simulink model "part1_WORKS"  (R2018b)
settings: Solver=FixedStepAuto  StartTime=0.0  StopTime=10.0  FixedStep=1e-3  RelTol=1e-3  EnableMultiTasking=on
undefined symbols (not defined in the file): A0, A1, D0, D1, D10, D11, D12, D13, D2, D3, D4, D5, D6, D7, D8, D9, PTA0, PTA1, PTA2, PTB2, PTB23, PTB3, PTB9, PTC16, PTC17, PTC2, PTC3, PTC4, PTD0, PTD1, PTD2, PTD3
libraries: frdmk64flib x26, xpcutilitieslib x9
settings Model: ExtModeTrigDuration=5  Creator=Buggs  LastModifiedBy=siddharthravichandran
settings OptimizationCC: PassReuseOutputArgsAs=Individual arguments  MaxStackSize=64
settings DebuggingCC: ParameterTunabilityLossMsg=error
settings HardwareCC: ProdBitPerPointer=32  ProdBitPerSizeT=32  ProdBitPerPtrDiffT=32  ProdLargestAtomicInteger=Long  ProdLargestAtomicFloat=Double  ProdWordSize=32  ProdHWDeviceType=ARM Compatible->ARM Cortex
settings SFSimCC: MATLABDynamicMemAlloc=off
settings RTWCC: SystemTargetFile=ert.tlc  HardwareBoard=NXP FRDM-K64F  TLCOptions="-aInlineSetEventsForThisBaseRateFcn=TLC_FALSE -aSuppressMultiTaskScheduler=TLC_FALSE  -aRateBasedStepFcn=0"  TemplateMakefile=ert_default_tmf  GenerateReport=on  Toolchain=GNU Tools for ARM Embedded Processors  IncludeHyperlinkInReport=on  LaunchReport=on  GenerateTraceInfo=on  GenerateTraceReport=on  GenerateTraceReportSl=on  GenerateTraceReportSf=on  GenerateTraceReportEml=on
settings CodeAppCC: ForceParamTrailComments=on  IgnoreCustomStorageClasses=off  OperatorAnnotations=on  SimulinkDataObjDesc=on  SFDataObjDesc=on  InsertBlockDesc=on

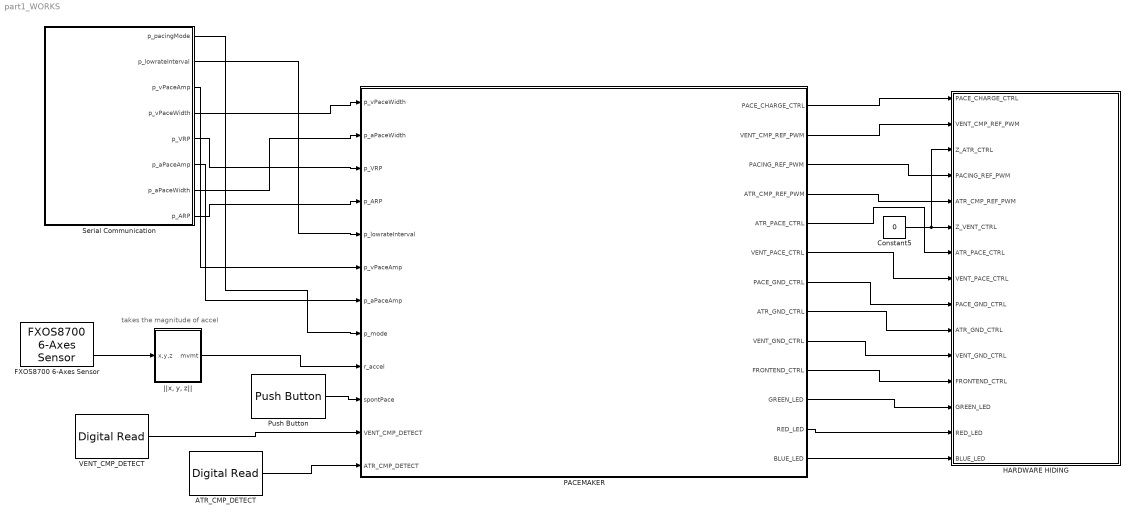
== system part1_WORKS ==
  note: takes the magnitude of accel
  ATR_CMP_DETECT : frdmk64flib/Digital Read  Whichpin=PTC16 (D0)  SampleTime=-1
      settings: SourceProductName=Simulink Coder Support Package for NXP FRDM-K64F Board
  Constant5 : Constant  Value=0  OutDataTypeStr=boolean
  FXOS8700 6-Axes Sensor : frdmk64flib/FXOS8700 6-Axes Sensor  Activesensor=Accelerometer and Magnetometer  ODR=800Hz  HybridODR=400Hz  Accelfullrange=-4g to +4g  SampleTime=-1
      settings: SourceProductName=Simulink Coder Support Package for NXP FRDM-K64F Board
  "HARDWARE HIDING " : Subsystem
  PACEMAKER : Stateflow chart  TreatAsAtomicUnit=on
  Push Button : frdmk64flib/Push Button  Whichswitch=SW2  SampleTime1=-1
      settings: SourceProductName=Simulink Coder Support Package for NXP FRDM-K64F Board
  Serial Communication : Subsystem
  VENT_CMP_DETECT : frdmk64flib/Digital Read  Whichpin=PTC17 (D1)  SampleTime=-1
      settings: SourceProductName=Simulink Coder Support Package for NXP FRDM-K64F Board
  "||x, y, z||" : Subsystem
  wires:
  FXOS8700 6-Axes Sensor/2 -> "||x, y, z||"/1(x,y,z)
  "||x, y, z||"/1(mvmt) -> PACEMAKER/9(r_accel)
  Serial Communication/2(p_lowrateInterval) -> PACEMAKER/5(p_lowrateInterval)
  Serial Communication/1(p_pacingMode) -> PACEMAKER/8(p_mode)
  Push Button/1 -> PACEMAKER/10(spontPace)
  VENT_CMP_DETECT/1 -> PACEMAKER/11(VENT_CMP_DETECT)
  ATR_CMP_DETECT/1 -> PACEMAKER/12(ATR_CMP_DETECT)
  PACEMAKER/11(GREEN_LED) -> "HARDWARE HIDING "/13(GREEN_LED)
  PACEMAKER/10(FRONTEND_CTRL) -> "HARDWARE HIDING "/12(FRONTEND_CTRL)
  PACEMAKER/4(ATR_CMP_REF_PWM) -> "HARDWARE HIDING "/5(ATR_CMP_REF_PWM)
  Constant5/1 -> "HARDWARE HIDING "/3(Z_ATR_CTRL), "HARDWARE HIDING "/6(Z_VENT_CTRL)
  PACEMAKER/1(PACE_CHARGE_CTRL) -> "HARDWARE HIDING "/1(PACE_CHARGE_CTRL)
  PACEMAKER/2(VENT_CMP_REF_PWM) -> "HARDWARE HIDING "/2(VENT_CMP_REF_PWM)
  PACEMAKER/7(PACE_GND_CTRL) -> "HARDWARE HIDING "/9(PACE_GND_CTRL)
  PACEMAKER/9(VENT_GND_CTRL) -> "HARDWARE HIDING "/11(VENT_GND_CTRL)
  PACEMAKER/6(VENT_PACE_CTRL) -> "HARDWARE HIDING "/8(VENT_PACE_CTRL)
  PACEMAKER/8(ATR_GND_CTRL) -> "HARDWARE HIDING "/10(ATR_GND_CTRL)
  PACEMAKER/5(ATR_PACE_CTRL) -> "HARDWARE HIDING "/7(ATR_PACE_CTRL)
  PACEMAKER/3(PACING_REF_PWM) -> "HARDWARE HIDING "/4(PACING_REF_PWM)
  PACEMAKER/12(RED_LED) -> "HARDWARE HIDING "/14(RED_LED)
  PACEMAKER/13(BLUE_LED) -> "HARDWARE HIDING "/15(BLUE_LED)
  Serial Communication/5(p_VRP) -> PACEMAKER/3(p_VRP)
  Serial Communication/8(p_ARP) -> PACEMAKER/4(p_ARP)
  Serial Communication/4(p_vPaceWidth) -> PACEMAKER/1(p_vPaceWidth)
  Serial Communication/7(p_aPaceWidth) -> PACEMAKER/2(p_aPaceWidth)
  Serial Communication/3(p_vPaceAmp) -> PACEMAKER/6(p_vPaceAmp)
  Serial Communication/6(p_aPaceAmp) -> PACEMAKER/7(p_aPaceAmp)

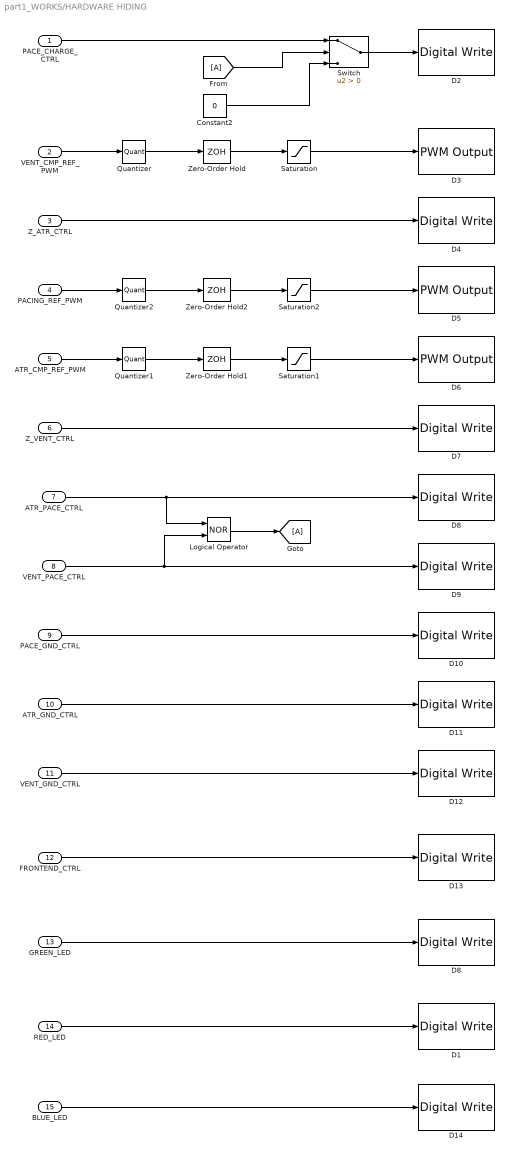
== system part1_WORKS/HARDWARE HIDING  ==
  PACE_CHARGE_CTRL : Inport  OutDataTypeStr=boolean
  VENT_CMP_REF_PWM : Inport  Port=2  OutDataTypeStr=double
  Z_ATR_CTRL : Inport  Port=3  OutDataTypeStr=boolean
  PACING_REF_PWM : Inport  Port=4  OutDataTypeStr=double
  ATR_CMP_REF_PWM : Inport  Port=5  OutDataTypeStr=double
  Z_VENT_CTRL : Inport  Port=6  OutDataTypeStr=boolean
  ATR_PACE_CTRL : Inport  Port=7  OutDataTypeStr=boolean
  VENT_PACE_CTRL : Inport  Port=8  OutDataTypeStr=boolean
  PACE_GND_CTRL : Inport  Port=9  OutDataTypeStr=boolean
  ATR_GND_CTRL : Inport  Port=10  OutDataTypeStr=boolean
  VENT_GND_CTRL : Inport  Port=11  OutDataTypeStr=boolean
  FRONTEND_CTRL : Inport  Port=12  OutDataTypeStr=boolean
  GREEN_LED : Inport  Port=13  OutDataTypeStr=boolean
  RED_LED : Inport  Port=14  OutDataTypeStr=boolean
  BLUE_LED : Inport  Port=15  OutDataTypeStr=boolean
  Constant2 : Constant  Value=0  OutDataTypeStr=boolean
  D1 : frdmk64flib/Digital Write  Whichpin=RED_LED
      settings: SourceProductName=Simulink Coder Support Package for NXP FRDM-K64F Board
  D10 : frdmk64flib/Digital Write  Whichpin=PTD0 (D10)
      settings: SourceProductName=Simulink Coder Support Package for NXP FRDM-K64F Board
  D11 : frdmk64flib/Digital Write  Whichpin=PTD2 (D11)
      settings: SourceProductName=Simulink Coder Support Package for NXP FRDM-K64F Board
  D12 : frdmk64flib/Digital Write  Whichpin=PTD3 (D12)
      settings: SourceProductName=Simulink Coder Support Package for NXP FRDM-K64F Board
  D13 : frdmk64flib/Digital Write  Whichpin=PTD1 (D13)
      settings: SourceProductName=Simulink Coder Support Package for NXP FRDM-K64F Board
  D14 : frdmk64flib/Digital Write  Whichpin=BLUE_LED
      settings: SourceProductName=Simulink Coder Support Package for NXP FRDM-K64F Board
  D2 : frdmk64flib/Digital Write  Whichpin=PTB9 (D2)
      settings: SourceProductName=Simulink Coder Support Package for NXP FRDM-K64F Board
  D3 : frdmk64flib/PWM Output  Whichpin=PTA1 (D3)  InitialFrequency=916  InitialDutyCycle=0
      settings: SourceProductName=Simulink Coder Support Package for NXP FRDM-K64F Board
  D4 : frdmk64flib/Digital Write  Whichpin=PTB23 (D4)
      settings: SourceProductName=Simulink Coder Support Package for NXP FRDM-K64F Board
  D5 : frdmk64flib/PWM Output  Whichpin=PTA2 (D5)  InitialFrequency=916  InitialDutyCycle=0
      settings: SourceProductName=Simulink Coder Support Package for NXP FRDM-K64F Board
  D6 : frdmk64flib/PWM Output  Whichpin=PTC2 (D6)  InitialFrequency=916  InitialDutyCycle=0
      settings: SourceProductName=Simulink Coder Support Package for NXP FRDM-K64F Board
  D7 : frdmk64flib/Digital Write  Whichpin=PTC3 (D7)
      settings: SourceProductName=Simulink Coder Support Package for NXP FRDM-K64F Board
  D8 : frdmk64flib/Digital Write  Whichpin=GREEN_LED
      settings: SourceProductName=Simulink Coder Support Package for NXP FRDM-K64F Board
  "D8 " : frdmk64flib/Digital Write  Whichpin=PTA0 (D8)
      settings: SourceProductName=Simulink Coder Support Package for NXP FRDM-K64F Board
  D9 : frdmk64flib/Digital Write  Whichpin=PTC4 (D9)
      settings: SourceProductName=Simulink Coder Support Package for NXP FRDM-K64F Board
  Logical Operator : Logic  Operator=NOR  AllPortsSameDT=off  OutDataTypeStr=boolean
  Quantizer : Quantizer  QuantizationInterval=0.01
  Quantizer1 : Quantizer  QuantizationInterval=0.01
  Quantizer2 : Quantizer  QuantizationInterval=0.01
  Saturation : Saturate  UpperLimit=100  LowerLimit=0
  Saturation1 : Saturate  UpperLimit=100  LowerLimit=0
  Saturation2 : Saturate  UpperLimit=100  LowerLimit=0
  Switch : Switch  Criteria=u2 > Threshold
  Zero-Order Hold : ZeroOrderHold  SampleTime=0.01
  Zero-Order Hold1 : ZeroOrderHold  SampleTime=0.01
  Zero-Order Hold2 : ZeroOrderHold  SampleTime=0.01
  wires:
  Z_ATR_CTRL/1 -> D4/1
  Z_VENT_CTRL/1 -> D7/1
  VENT_PACE_CTRL/1 -> D9/1, Logical Operator/2
  PACE_GND_CTRL/1 -> D10/1
  ATR_GND_CTRL/1 -> D11/1
  VENT_GND_CTRL/1 -> D12/1
  FRONTEND_CTRL/1 -> D13/1
  ATR_PACE_CTRL/1 -> "D8 "/1, Logical Operator/1
  Switch/1 -> D2/1
  PACE_CHARGE_CTRL/1 -> Switch/1
  Constant2/1 -> Switch/3
  VENT_CMP_REF_PWM/1 -> Quantizer/1
  Quantizer/1 -> Zero-Order Hold/1
  Quantizer1/1 -> Zero-Order Hold1/1
  Zero-Order Hold1/1 -> Saturation1/1
  Saturation1/1 -> D6/1
  ATR_CMP_REF_PWM/1 -> Quantizer1/1
  Zero-Order Hold2/1 -> Saturation2/1
  Saturation2/1 -> D5/1
  Quantizer2/1 -> Zero-Order Hold2/1
  PACING_REF_PWM/1 -> Quantizer2/1
  [A] -> Switch/2
  Logical Operator/1 -> [A]
  Saturation/1 -> D3/1
  Zero-Order Hold/1 -> Saturation/1
  GREEN_LED/1 -> D8/1
  RED_LED/1 -> D1/1
  BLUE_LED/1 -> D14/1

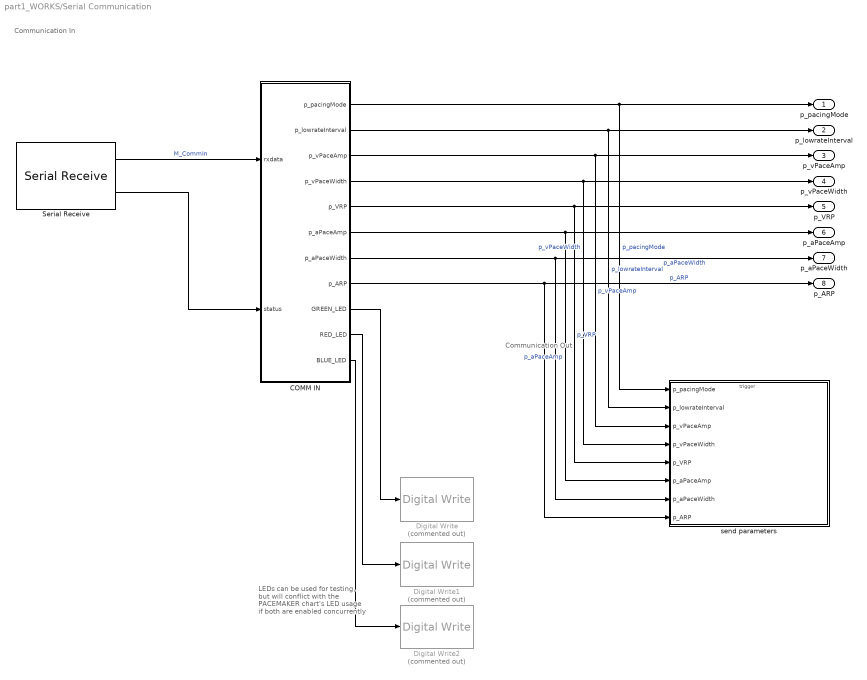
== system part1_WORKS/Serial Communication ==
  note: LEDs can be used for testing,
      | but will conflict with the
      | PACEMAKER chart's LED
      | usage if both are enabled
      | concurrently
  note: Communication Out
  note: Communication In
  COMM IN : Stateflow chart  TreatAsAtomicUnit=on
  Digital Write : frdmk64flib/Digital Write  Commented=on  Whichpin=GREEN_LED
      settings: SourceProductName=Simulink Coder Support Package for NXP FRDM-K64F Board
  Digital Write1 : frdmk64flib/Digital Write  Commented=on  Whichpin=RED_LED
      settings: SourceProductName=Simulink Coder Support Package for NXP FRDM-K64F Board
  Digital Write2 : frdmk64flib/Digital Write  Commented=on  Whichpin=BLUE_LED
      settings: SourceProductName=Simulink Coder Support Package for NXP FRDM-K64F Board
  Serial Receive : frdmk64flib/Serial Receive  SCIModule=0  Baudrate=uint32(9600)  Parity=None  StopBits=1  HardwareFlowControl=None  ByteOrder=LittleEndian  DataType=uint8  DataLength=22  BlockingMode=off  OutputStatus=on  SampleTime=-1
      settings: SourceProductName=Simulink Coder Support Package for NXP FRDM-K64F Board
  send parameters : Subsystem
  p_pacingMode : Outport
  p_lowrateInterval : Outport  Port=2
  p_vPaceAmp : Outport  Port=3
  p_vPaceWidth : Outport  Port=4
  p_VRP : Outport  Port=5
  p_aPaceAmp : Outport  Port=6
  p_aPaceWidth : Outport  Port=7
  p_ARP : Outport  Port=8
  wires:
  COMM IN/5(p_VRP) -> send parameters/5(p_VRP), p_VRP/1  "p_VRP"
  COMM IN/1(p_pacingMode) -> send parameters/1(p_pacingMode), p_pacingMode/1  "p_pacingMode"
  COMM IN/7(p_aPaceWidth) -> send parameters/7(p_aPaceWidth), p_aPaceWidth/1  "p_aPaceWidth"
  COMM IN/4(p_vPaceWidth) -> send parameters/4(p_vPaceWidth), p_vPaceWidth/1  "p_vPaceWidth"
  COMM IN/8(p_ARP) -> send parameters/8(p_ARP), p_ARP/1  "p_ARP"
  COMM IN/6(p_aPaceAmp) -> send parameters/6(p_aPaceAmp), p_aPaceAmp/1  "p_aPaceAmp"
  COMM IN/3(p_vPaceAmp) -> send parameters/3(p_vPaceAmp), p_vPaceAmp/1  "p_vPaceAmp"
  COMM IN/2(p_lowrateInterval) -> send parameters/2(p_lowrateInterval), p_lowrateInterval/1  "p_lowrateInterval"
  COMM IN/10(RED_LED) -> Digital Write1/1
  COMM IN/9(GREEN_LED) -> Digital Write/1
  COMM IN/11(BLUE_LED) -> Digital Write2/1
  Serial Receive/1 -> COMM IN/1(rxdata)  "M_CommIn"
  Serial Receive/2 -> COMM IN/2(status)

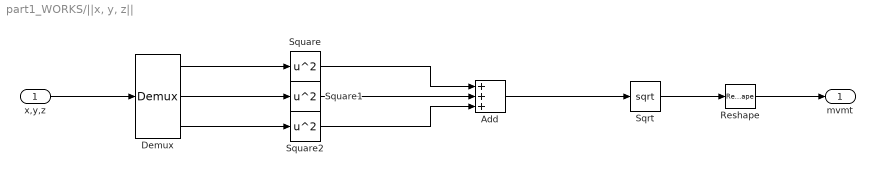
== system part1_WORKS/||x, y, z|| ==
  x,y,z : Inport
  Add : Sum  Inputs=+++
  Demux : Demux  Outputs=3
  Reshape : Reshape  OutputDimensions=[1]
  Sqrt : Sqrt  SaturateOnIntegerOverflow=on
  Square : Math  Operator=square  SaturateOnIntegerOverflow=on
  Square1 : Math  Operator=square  SaturateOnIntegerOverflow=on
  Square2 : Math  Operator=square  SaturateOnIntegerOverflow=on
  mvmt : Outport
  wires:
  x,y,z/1 -> Demux/1
  Sqrt/1 -> Reshape/1
  Square/1 -> Add/1
  Square1/1 -> Add/2
  Demux/3 -> Square2/1
  Add/1 -> Sqrt/1
  Demux/2 -> Square1/1
  Square2/1 -> Add/3
  Demux/1 -> Square/1
  Reshape/1 -> mvmt/1

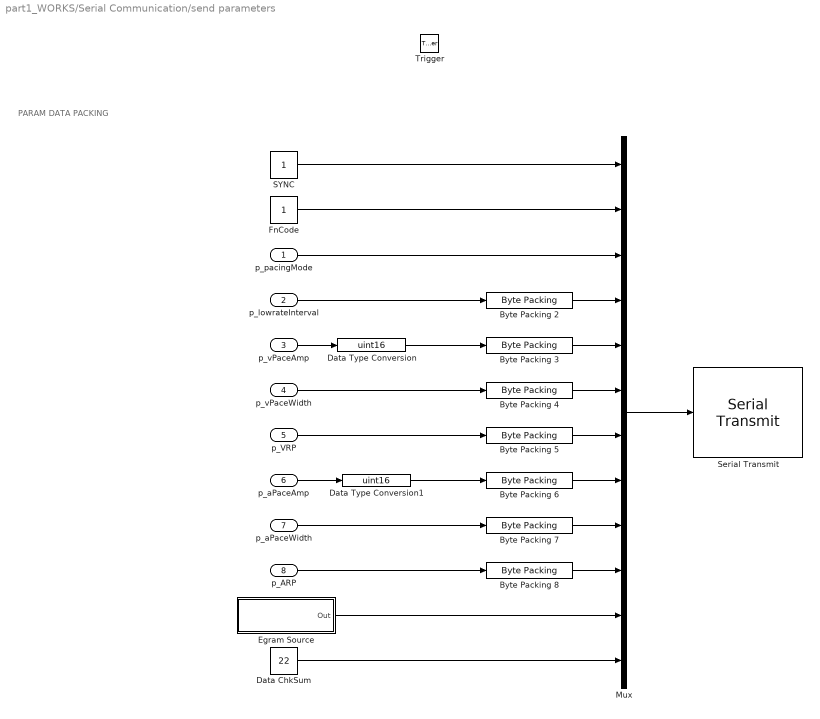
== system part1_WORKS/Serial Communication/send parameters ==
  note: PARAM DATA PACKING
  p_pacingMode : Inport
  p_lowrateInterval : Inport  Port=2
  p_vPaceAmp : Inport  Port=3
  p_vPaceWidth : Inport  Port=4
  p_VRP : Inport  Port=5
  p_aPaceAmp : Inport  Port=6
  p_aPaceWidth : Inport  Port=7
  p_ARP : Inport  Port=8
  Trigger : TriggerPort  TriggerType=function-call  IsSimulinkFunction=on  FunctionName=send_data  VariantControl=Variant  PortDimensions=1
      settings: GeneratePreprocessorConditionals=on
  Byte Packing {2..8} (7 alike) : xpcutilitieslib/Byte Packing   MaskPackedDataType=uint8  MaskUnpackedDataTypes={'uint16'}  MaskAlignment=1
  Data ChkSum : Constant  Value=22  OutDataTypeStr=uint8
  Data Type Conversion : DataTypeConversion  OutDataTypeStr=uint16
  Data Type Conversion1 : DataTypeConversion  OutDataTypeStr=uint16
  Egram Source : Subsystem
  FnCode : Constant  OutDataTypeStr=uint8
  Mux : Mux  Inputs=12
  SYNC : Constant  OutDataTypeStr=uint8
  Serial Transmit : frdmk64flib/Serial Transmit  SCIModule=0  Baudrate=uint32(9600)  Parity=None  StopBits=1  HardwareFlowControl=None  ByteOrder=LittleEndian  BlockingMode=on  OutputStatus=off
      settings: SourceProductName=Simulink Coder Support Package for NXP FRDM-K64F Board
  wires:
  p_lowrateInterval/1 -> Byte Packing 2/1
  p_vPaceAmp/1 -> Data Type Conversion/1
  p_VRP/1 -> Byte Packing 5/1
  p_aPaceAmp/1 -> Data Type Conversion1/1
  p_ARP/1 -> Byte Packing 8/1
  Byte Packing 8/1 -> Mux/10
  Byte Packing 7/1 -> Mux/9
  Byte Packing 6/1 -> Mux/8
  Byte Packing 5/1 -> Mux/7
  Byte Packing 4/1 -> Mux/6
  Byte Packing 3/1 -> Mux/5
  Byte Packing 2/1 -> Mux/4
  p_pacingMode/1 -> Mux/3
  FnCode/1 -> Mux/2
  SYNC/1 -> Mux/1
  Data ChkSum/1 -> Mux/12
  Egram Source/1(Out) -> Mux/11
  Mux/1 -> Serial Transmit/1
  p_vPaceWidth/1 -> Byte Packing 4/1
  p_aPaceWidth/1 -> Byte Packing 7/1
  Data Type Conversion/1 -> Byte Packing 3/1
  Data Type Conversion1/1 -> Byte Packing 6/1

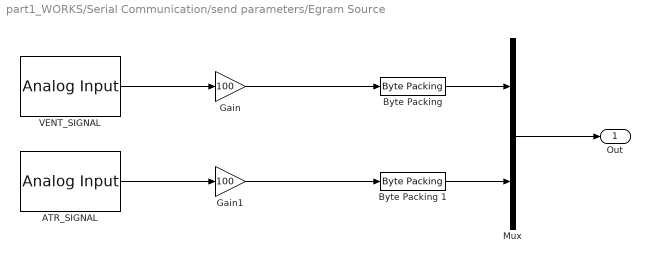
== system part1_WORKS/Serial Communication/send parameters/Egram Source ==
  ATR_SIGNAL : frdmk64flib/Analog Input  Whichpin=PTB2 (A0)  SampleTime=-1
      settings: SourceProductName=Simulink Coder Support Package for NXP FRDM-K64F Board
  "Byte Packing " : xpcutilitieslib/Byte Packing   MaskPackedDataType=uint8  MaskUnpackedDataTypes={'int16'}  MaskAlignment=1
  Byte Packing 1 : xpcutilitieslib/Byte Packing   MaskPackedDataType=uint8  MaskUnpackedDataTypes={'int16'}  MaskAlignment=1
  Gain : Gain  Gain=100  OutDataTypeStr=int16
  Gain1 : Gain  Gain=100  OutDataTypeStr=int16  RndMeth=Round
  Mux : Mux  Inputs=2
  VENT_SIGNAL : frdmk64flib/Analog Input  Whichpin=PTB3 (A1)  SampleTime=-1
      settings: SourceProductName=Simulink Coder Support Package for NXP FRDM-K64F Board
  Out : Outport
  wires:
  VENT_SIGNAL/1 -> Gain/1
  ATR_SIGNAL/1 -> Gain1/1
  Byte Packing 1/1 -> Mux/2
  Gain1/1 -> Byte Packing 1/1
  Mux/1 -> Out/1
  "Byte Packing "/1 -> Mux/1
  Gain/1 -> "Byte Packing "/1

== stateflow chart part1_WORKS/Serial Communication/COMM IN ==
  settings: executeAtInitialization=1
  state PROG_PARAMS
    %sets given vals
    entry:
    p_pacingMode(1)=rxdata(3);
    p_lowrateInterval(1)=typecast(rxdata(4:5),'uint16');
    p_vPaceAmp(1)=cast(typecast(rxdata(6:7),'uint16'),'double');
    p_vPaceWidth(1)=typecast(rxdata(8:9),'uint16');
    p_VRP(1)=typecast(rxdata(10:11),'uint16');
    p_aPaceAmp(1)=cast(typecast(rxdata(12:13),'uint16'),'double');
    p_aPaceWidth(1)=typecast(rxdata(14:15),'int16');
    p_ARP(1)=typecast(rxdata(16:17),'uint16');
    RED_LED = true;
    GREEN_LED = false;
    BLUE_LED = false;
  state INITIAL
    entry:
    p_pacingMode = uint8(0);
    p_lowrateInterval = uint16(1000);
    p_vPaceAmp = double(60);
    p_vPaceWidth = uint16(100); %needs to be changed
    p_VRP = uint16(320);
    p_aPaceAmp = double(60);
    p_aPaceWidth = uint16(100); %need to be changed
    p_ARP = uint16(320);
  note: SYNC == 1
  note: status == 0
  note: Data ChkSum == 22
  state STANDBY
    %entry:
    %send_data();
    entry: RED_LED=false;
    BLUE_LED=true;
    GREEN_LED=false;
  state ECHO_PARAM
    entry:
    send_data();
    RED_LED = false;
    GREEN_LED = true;
    BLUE_LED = false;
  note: make sure to store info as local value and remove SEND_EGRAM
  PROG_PARAMS -> STANDBY : after(500,msec)
  (junction 105) -> PROG_PARAMS [order 2] : [rxdata(2)==1]
  (junction 105) -> STANDBY [order 3]
  (default) -> INITIAL
  STANDBY -> (junction 105) : [rxdata(1)==1 && status == 0 && rxdata(length(rxdata))==22]
  (junction 105) -> ECHO_PARAM [order 1] : [rxdata(2)==0]
  INITIAL -> STANDBY
  ECHO_PARAM -> STANDBY : after(500,msec)
  data: rxdata input uint8; status input uint8; p_pacingMode output uint8; p_lowrateInterval output uint16; p_vPaceAmp output double; p_vPaceWidth output uint16; p_VRP output uint16; p_aPaceAmp output double; p_aPaceWidth output uint16; p_ARP output uint16; GREEN_LED output boolean; RED_LED output boolean; BLUE_LED output boolean

== stateflow chart part1_WORKS/PACEMAKER ==
  state VVIR
    state PACE [parallel]
      settings: executionOrder=1
      state CHARGE_BLOCK
        entry:
        PACE_CHARGE_CTRL=false;
        VENT_PACE_CTRL=true;
        VENT_GND_CTRL=false;
        GREEN_LED = true;
        RED_LED = false;
        l_paced = true;
        l_sense = false;
      state DISCHARGE_CHARGE
        entry:
        PACING_REF_PWM=p_vPaceAmp;
        PACE_CHARGE_CTRL=true;
        VENT_PACE_CTRL=false;
        VENT_GND_CTRL=true;
        PACE_GND_CTRL=true;
        GREEN_LED = false;
        RED_LED = false;
      state INIT_LRL
        entry:
        l_lowrateInterval=p_lowrateInterval;
        l_setpoint = l_lowrateInterval;
        VENT_CMP_REF_PWM = 60;
        ATR_CMP_REF_PWM = 60;
        FRONTEND_CTRL= true;
        l_paced = false;
      state BLANK
        entry:
        RED_LED=true;
        l_sense=false;
        l_paced=true;
      note: INIT_LRL incorporates the local variables required for rate-adaptivity
          | and for inhibition
      VVIR.PACE.DISCHARGE_CHARGE -> VVIR.PACE.CHARGE_BLOCK [order 1] : after(l_lowrateInterval-p_vPaceWidth,msec)
      VVIR.PACE.CHARGE_BLOCK -> VVIR.PACE.DISCHARGE_CHARGE : after(p_vPaceWidth,msec)
      VVIR.PACE.BLANK -> VVIR.PACE.CHARGE_BLOCK [order 1] : after(l_lowrateInterval,msec)
      VVIR.PACE.INIT_LRL -> VVIR.PACE.DISCHARGE_CHARGE
      VVIR.PACE.DISCHARGE_CHARGE -> VVIR.PACE.BLANK [order 2] : [l_sense==true && VENT_CMP_DETECT==true]
      VVIR.PACE.BLANK -> VVIR.PACE.BLANK [order 2] : [l_sense==true && VENT_CMP_DETECT==true]
      (default) -> VVIR.PACE.INIT_LRL
    state SETTER [parallel]
      settings: executionOrder=2
      state INC_INT
        entry:
        l_lowrateInterval=l_lowrateInterval+10;
      state CHECK_SET
      state STAY
      state DEC_INT
        entry:
        l_lowrateInterval=l_lowrateInterval-10;
      (default) -> VVIR.SETTER.CHECK_SET
      VVIR.SETTER.INC_INT -> VVIR.SETTER.CHECK_SET : after(100,msec)
      (junction 149) -> VVIR.SETTER.INC_INT [order 2] : [l_setpoint-10>l_lowrateInterval]
      VVIR.SETTER.CHECK_SET -> (junction 149) [order 1] : [l_setpoint+10>=l_lowrateInterval]
      (junction 149) -> VVIR.SETTER.STAY [order 1] : [l_setpoint-10<=l_lowrateInterval]
      VVIR.SETTER.DEC_INT -> VVIR.SETTER.CHECK_SET : after(100,msec)
      VVIR.SETTER.STAY -> VVIR.SETTER.CHECK_SET : after(100,msec)
      VVIR.SETTER.CHECK_SET -> VVIR.SETTER.DEC_INT [order 2] : [l_setpoint+10<l_lowrateInterval]
    note: rate adaptivity changes l_lowrateInterval, so the PACE state needs no significant change
    note: COUNTER, TIMER, and SETTER are identical to VOOR
    state COUNTER [parallel]
      settings: executionOrder=3
      state BLANK
      state ADD_COUNT
        entry:
        l_status=l_status+1;
      (default) -> VVIR.COUNTER.BLANK
      VVIR.COUNTER.BLANK -> VVIR.COUNTER.ADD_COUNT : [r_accel>=2]
      VVIR.COUNTER.ADD_COUNT -> VVIR.COUNTER.BLANK : after(200,msec)
    note: The rate-adaptive and pace inhibition subsystems are designed
        | to work independently or together and can be run in parallel to
        | achieve both requirements at the same time.
    state TIMER [parallel]
      settings: executionOrder=4
      state PICK_ACTIVITY
      state REST
        entry:
        l_setpoint=1000;
      state SPRINT
        entry:
        l_setpoint=330;
      state F_JOG
        entry:
        l_setpoint=425;
      state F_WALK
        entry:
        l_setpoint=600;
      state RESET_TIME
        entry:
        l_status=0;
      state RUN
        entry:
        l_setpoint=375;
      state S_JOG
        entry:
        l_setpoint=500;
      state S_WALK
        entry:
        l_setpoint=750;
      state END_TIME
      VVIR.TIMER.RESET_TIME -> VVIR.TIMER.PICK_ACTIVITY : after(3000,msec)
      VVIR.TIMER.PICK_ACTIVITY -> VVIR.TIMER.SPRINT [order 1] : [l_status>=7]
      VVIR.TIMER.PICK_ACTIVITY -> VVIR.TIMER.RUN [order 2] : [l_status>=6]
      VVIR.TIMER.PICK_ACTIVITY -> VVIR.TIMER.F_JOG [order 3] : [l_status>=5]
      VVIR.TIMER.PICK_ACTIVITY -> VVIR.TIMER.S_JOG [order 4] : [l_status>=4]
      VVIR.TIMER.PICK_ACTIVITY -> VVIR.TIMER.F_WALK [order 5] : [l_status>=3]
      VVIR.TIMER.PICK_ACTIVITY -> VVIR.TIMER.S_WALK [order 6] : [l_status>=2]
      VVIR.TIMER.PICK_ACTIVITY -> VVIR.TIMER.REST [order 7] : [l_status<2]
      (default) -> VVIR.TIMER.RESET_TIME
      VVIR.TIMER.REST -> VVIR.TIMER.END_TIME
      VVIR.TIMER.SPRINT -> VVIR.TIMER.END_TIME
      VVIR.TIMER.F_JOG -> VVIR.TIMER.END_TIME
      VVIR.TIMER.F_WALK -> VVIR.TIMER.END_TIME
      VVIR.TIMER.END_TIME -> VVIR.TIMER.RESET_TIME
      VVIR.TIMER.RUN -> VVIR.TIMER.END_TIME
      VVIR.TIMER.S_JOG -> VVIR.TIMER.END_TIME
      VVIR.TIMER.S_WALK -> VVIR.TIMER.END_TIME
    state REFRACTORY [parallel]
      settings: executionOrder=5
      state START
      state PACED
        entry:
        l_paced=false;
      state ALLOW_SENSE
        entry:
        l_sense=true;
      VVIR.REFRACTORY.ALLOW_SENSE -> VVIR.REFRACTORY.START
      VVIR.REFRACTORY.START -> VVIR.REFRACTORY.PACED : [l_paced==true]
      VVIR.REFRACTORY.PACED -> VVIR.REFRACTORY.ALLOW_SENSE : after(p_VRP, msec)
    note: REFRACTORY is dentical to VVI
    (default) -> VVIR.REFRACTORY.START
  note: mode controller resets sensing, and turns on blue light
      | while within the mode.
      | Exits when p_mode reaches a valid state
  state VOO
    note: sets switches to charge capacitor
    note: sets switches to pace the heart
    note: determines BPM of the paces
    state CHARGE_BLOCK
      entry:
      PACE_CHARGE_CTRL=false;
      VENT_PACE_CTRL=true;
      VENT_GND_CTRL=false;
    state DISCHARGE_CHARGE
      entry:
      PACING_REF_PWM=p_vPaceAmp;
      PACE_CHARGE_CTRL=true;
      VENT_PACE_CTRL=false;
      VENT_GND_CTRL=true;
      PACE_GND_CTRL=true;
    note: determines pace width
    VOO.DISCHARGE_CHARGE -> VOO.CHARGE_BLOCK : after(p_lowrateInterval-p_vPaceWidth,msec)
    (default) -> VOO.DISCHARGE_CHARGE
    VOO.CHARGE_BLOCK -> VOO.DISCHARGE_CHARGE : after(p_vPaceWidth,msec)
  state CHOOSE_MODE
    entry:
    GREEN_LED=false;
    RED_LED=false;
    BLUE_LED=true;
    FRONTEND_CTRL=false;
    exit:
    BLUE_LED=false
  state AOO
    note: structure is identical to VOO (above), except for atrial variables
    state CHARGE_BLOCK
      entry:
      PACE_CHARGE_CTRL=false;
      ATR_PACE_CTRL=true;
      ATR_GND_CTRL=false;
    state DISCHARGE_CHARGE
      entry:
      PACING_REF_PWM=p_aPaceAmp;
      PACE_CHARGE_CTRL=true;
      ATR_PACE_CTRL=false;
      ATR_GND_CTRL=true;
      PACE_GND_CTRL=true;
    AOO.DISCHARGE_CHARGE -> AOO.CHARGE_BLOCK : after(p_lowrateInterval-p_aPaceWidth,msec)
    (default) -> AOO.DISCHARGE_CHARGE
    AOO.CHARGE_BLOCK -> AOO.DISCHARGE_CHARGE : after(p_aPaceWidth,msec)
  state VVI
    state PACE [parallel]
      settings: executionOrder=1
      state DISCHARGE_CHARGE
        entry:
        PACING_REF_PWM=p_vPaceAmp;
        PACE_CHARGE_CTRL=true;
        VENT_PACE_CTRL=false;
        VENT_GND_CTRL=true;
        PACE_GND_CTRL=true;
        GREEN_LED = false;
        RED_LED = false;
      state CHARGE_BLOCK
        entry:
        PACE_CHARGE_CTRL=false;
        VENT_PACE_CTRL=true;
        VENT_GND_CTRL=false;
        GREEN_LED = true;
        l_paced = true;
        l_sense = false;
      note: if a natural pace is detected,
          | and sensing is allowed
      state INIT_LRL
        entry:
        FRONTEND_CTRL= true;
        l_paced = false;
        l_sense = false;
        VENT_CMP_REF_PWM = 60;
        ATR_CMP_REF_PWM = 60;
      note: if no natural beat for lowrateInterval,
          | back to regular pacing
      state BLANK
        entry:
        RED_LED=true;
        l_sense=false;
        l_paced=true;
      note: sensing activated,
          | intial local variables are set,
          | reference voltages set
      note: set RED_LED to indicate inhibition
      note: every time a pacing state is entered, (BLANK or CHARGE_BLOCK),
          | l_sense is set to false and l_paced to true
      VVI.PACE.DISCHARGE_CHARGE -> VVI.PACE.CHARGE_BLOCK [order 1] : after(p_lowrateInterval-p_vPaceWidth,msec)
      VVI.PACE.CHARGE_BLOCK -> VVI.PACE.DISCHARGE_CHARGE : after(p_vPaceWidth,msec)
      VVI.PACE.BLANK -> VVI.PACE.CHARGE_BLOCK [order 1] : after(p_lowrateInterval,msec)
      VVI.PACE.INIT_LRL -> VVI.PACE.DISCHARGE_CHARGE
      VVI.PACE.DISCHARGE_CHARGE -> VVI.PACE.BLANK [order 2] : [l_sense==true && VENT_CMP_DETECT==true]
      VVI.PACE.BLANK -> VVI.PACE.BLANK [order 2] : [l_sense==true && VENT_CMP_DETECT==true]
      (default) -> VVI.PACE.INIT_LRL
    state REFRACTORY [parallel]
      settings: executionOrder=2
      state START
      state PACED
        entry:
        l_paced=false;
      state ALLOW_SENSE
        entry:
        l_sense=true;
      note: if the heart was paced, wait for refractory period before allowing sensing
          | (l_sense is set to false in pacing states)
      (default) -> VVI.REFRACTORY.START
      VVI.REFRACTORY.ALLOW_SENSE -> VVI.REFRACTORY.START
      VVI.REFRACTORY.START -> VVI.REFRACTORY.PACED : [l_paced==true]
      VVI.REFRACTORY.PACED -> VVI.REFRACTORY.ALLOW_SENSE : after(p_VRP, msec)
    note: loop state if multiple natural paces
  state AAIR
    state PACE [parallel]
      settings: executionOrder=1
      state CHARGE_BLOCK
        entry:
        PACE_CHARGE_CTRL=false;
        ATR_PACE_CTRL=true;
        ATR_GND_CTRL=false;
        GREEN_LED = true;
        l_paced = true;
        l_sense = false;
      state DISCHARGE_CHARGE
        entry:
        PACING_REF_PWM=p_aPaceAmp;
        PACE_CHARGE_CTRL=true;
        ATR_PACE_CTRL=false;
        ATR_GND_CTRL=true;
        PACE_GND_CTRL=true;
        GREEN_LED = false;
        RED_LED = false;
      state INIT_LRL
        entry:
        l_lowrateInterval=p_lowrateInterval;
        l_setpoint = l_lowrateInterval;
        VENT_CMP_REF_PWM = 60;
        ATR_CMP_REF_PWM = 60;
        FRONTEND_CTRL= true;
        l_paced = false;
      state BLANK
        entry:
        RED_LED=true;
        l_sense=false;
        l_paced=true;
      AAIR.PACE.DISCHARGE_CHARGE -> AAIR.PACE.CHARGE_BLOCK [order 1] : after(l_lowrateInterval-p_aPaceWidth,msec)
      AAIR.PACE.CHARGE_BLOCK -> AAIR.PACE.DISCHARGE_CHARGE : after(p_aPaceWidth,msec)
      AAIR.PACE.BLANK -> AAIR.PACE.CHARGE_BLOCK [order 1] : after(l_lowrateInterval,msec)
      AAIR.PACE.INIT_LRL -> AAIR.PACE.DISCHARGE_CHARGE
      AAIR.PACE.DISCHARGE_CHARGE -> AAIR.PACE.BLANK [order 2] : [l_sense==true && ATR_CMP_DETECT==true]
      AAIR.PACE.BLANK -> AAIR.PACE.BLANK [order 2] : [l_sense==true && ATR_CMP_DETECT==true]
    note: identical to VVIR (above) except atrial variables are used instead
    state SETTER [parallel]
      settings: executionOrder=2
      state INC_INT
        entry:
        l_lowrateInterval=l_lowrateInterval+10;
      state CHECK_SET
      state STAY
      state DEC_INT
        entry:
        l_lowrateInterval=l_lowrateInterval-10;
      (default) -> AAIR.SETTER.CHECK_SET
      AAIR.SETTER.INC_INT -> AAIR.SETTER.CHECK_SET : after(100,msec)
      (junction 481) -> AAIR.SETTER.INC_INT [order 2] : [l_setpoint-10>l_lowrateInterval]
      AAIR.SETTER.CHECK_SET -> (junction 481) [order 1] : [l_setpoint+10>=l_lowrateInterval]
      (junction 481) -> AAIR.SETTER.STAY [order 1] : [l_setpoint-10<=l_lowrateInterval]
      AAIR.SETTER.DEC_INT -> AAIR.SETTER.CHECK_SET : after(100,msec)
      AAIR.SETTER.STAY -> AAIR.SETTER.CHECK_SET : after(100,msec)
      AAIR.SETTER.CHECK_SET -> AAIR.SETTER.DEC_INT [order 2] : [l_setpoint+10<l_lowrateInterval]
    state REFRACTORY [parallel]
      settings: executionOrder=5
      state START
      state PACED
        entry:
        l_paced=false;
      state ALLOW_SENSE
        entry:
        l_sense=true;
      (default) -> AAIR.REFRACTORY.START
      AAIR.REFRACTORY.ALLOW_SENSE -> AAIR.REFRACTORY.START
      AAIR.REFRACTORY.START -> AAIR.REFRACTORY.PACED : [l_paced==true]
      AAIR.REFRACTORY.PACED -> AAIR.REFRACTORY.ALLOW_SENSE : after(p_ARP, msec)
    state TIMER [parallel]
      settings: executionOrder=4
      state PICK_ACTIVITY
      state REST
        entry:
        l_setpoint=1000;
      state SPRINT
        entry:
        l_setpoint=330;
      state F_JOG
        entry:
        l_setpoint=425;
      state F_WALK
        entry:
        l_setpoint=600;
      state RESET_TIME
        entry:
        l_status=0;
      state RUN
        entry:
        l_setpoint=375;
      state S_JOG
        entry:
        l_setpoint=500;
      state S_WALK
        entry:
        l_setpoint=750;
      state END_TIME
      AAIR.TIMER.RESET_TIME -> AAIR.TIMER.PICK_ACTIVITY : after(3000,msec)
      AAIR.TIMER.PICK_ACTIVITY -> AAIR.TIMER.SPRINT [order 1] : [l_status>=7]
      AAIR.TIMER.PICK_ACTIVITY -> AAIR.TIMER.RUN [order 2] : [l_status>=6]
      AAIR.TIMER.PICK_ACTIVITY -> AAIR.TIMER.F_JOG [order 3] : [l_status>=5]
      AAIR.TIMER.PICK_ACTIVITY -> AAIR.TIMER.S_JOG [order 4] : [l_status>=4]
      AAIR.TIMER.PICK_ACTIVITY -> AAIR.TIMER.F_WALK [order 5] : [l_status>=3]
      AAIR.TIMER.PICK_ACTIVITY -> AAIR.TIMER.S_WALK [order 6] : [l_status>=2]
      AAIR.TIMER.PICK_ACTIVITY -> AAIR.TIMER.REST [order 7] : [l_status<2]
      (default) -> AAIR.TIMER.RESET_TIME
      AAIR.TIMER.REST -> AAIR.TIMER.END_TIME
      AAIR.TIMER.SPRINT -> AAIR.TIMER.END_TIME
      AAIR.TIMER.F_JOG -> AAIR.TIMER.END_TIME
      AAIR.TIMER.F_WALK -> AAIR.TIMER.END_TIME
      AAIR.TIMER.END_TIME -> AAIR.TIMER.RESET_TIME
      AAIR.TIMER.RUN -> AAIR.TIMER.END_TIME
      AAIR.TIMER.S_JOG -> AAIR.TIMER.END_TIME
      AAIR.TIMER.S_WALK -> AAIR.TIMER.END_TIME
    state COUNTER [parallel]
      settings: executionOrder=3
      state BLANK
      state ADD_COUNT
        entry:
        l_status=l_status+1;
      (default) -> AAIR.COUNTER.BLANK
      AAIR.COUNTER.BLANK -> AAIR.COUNTER.ADD_COUNT : [r_accel>=2]
      AAIR.COUNTER.ADD_COUNT -> AAIR.COUNTER.BLANK : after(200,msec)
    (default) -> AAIR.PACE.INIT_LRL
  state AAI
    state REFRACTORY [parallel]
      settings: executionOrder=2
      state START
      state PACED
        entry:
        l_paced=false;
      state ALLOW_SENSE
        entry:
        l_sense=true;
      (default) -> AAI.REFRACTORY.START
      AAI.REFRACTORY.ALLOW_SENSE -> AAI.REFRACTORY.START
      AAI.REFRACTORY.START -> AAI.REFRACTORY.PACED : [l_paced==true]
      AAI.REFRACTORY.PACED -> AAI.REFRACTORY.ALLOW_SENSE : after(p_ARP, msec)
    note: structure is identical to VVI
        | (above), except for atrial variables
    state PACE [parallel]
      settings: executionOrder=1
      state DISCHARGE_CHARGE
        entry:
        PACING_REF_PWM=p_aPaceAmp;
        PACE_CHARGE_CTRL=true;
        ATR_PACE_CTRL=false;
        ATR_GND_CTRL=true;
        PACE_GND_CTRL=true;
        GREEN_LED = false;
        RED_LED = false;
      state CHARGE_BLOCK
        entry:
        PACE_CHARGE_CTRL=false;
        ATR_PACE_CTRL=true;
        ATR_GND_CTRL=false;
        GREEN_LED = true;
        l_paced = true;
        l_sense = false;
      state INIT_LRL
        entry:
        FRONTEND_CTRL= true;
        l_paced = false;
        l_sense = false;
        VENT_CMP_REF_PWM = 60;
        ATR_CMP_REF_PWM = 60;
      state BLANK
        entry:
        RED_LED=true;
        l_sense=false;
        l_paced=true;
      AAI.PACE.DISCHARGE_CHARGE -> AAI.PACE.CHARGE_BLOCK [order 1] : after(p_lowrateInterval-p_aPaceWidth,msec)
      AAI.PACE.CHARGE_BLOCK -> AAI.PACE.DISCHARGE_CHARGE : after(p_aPaceWidth,msec)
      AAI.PACE.BLANK -> AAI.PACE.CHARGE_BLOCK [order 1] : after(p_lowrateInterval,msec)
      AAI.PACE.INIT_LRL -> AAI.PACE.DISCHARGE_CHARGE
      AAI.PACE.DISCHARGE_CHARGE -> AAI.PACE.BLANK [order 2] : [l_sense==true && ATR_CMP_DETECT==true]
      AAI.PACE.BLANK -> AAI.PACE.BLANK [order 2] : [l_sense==true && ATR_CMP_DETECT==true]
      (default) -> AAI.PACE.INIT_LRL
  state VOOR
    state PACE [parallel]
      settings: executionOrder=1
      state DISCHARGE_CHARGE
        entry:
        PACING_REF_PWM=p_vPaceAmp;
        PACE_CHARGE_CTRL=true;
        VENT_PACE_CTRL=false;
        VENT_GND_CTRL=true;
        PACE_GND_CTRL=true;
        GREEN_LED = false;
      state CHARGE_BLOCK
        entry:
        PACE_CHARGE_CTRL=false;
        VENT_PACE_CTRL=true;
        VENT_GND_CTRL=false;
        GREEN_LED = true;
      state INIT_LRL
        entry:
        l_lowrateInterval=p_lowrateInterval;
        l_setpoint = l_lowrateInterval;
      note: structure of the CHARGE_BLOCK and DISCHARGE_CHARGE
          | are identical to VOO implementation.
      note: used to initialize local variables
      VOOR.PACE.DISCHARGE_CHARGE -> VOOR.PACE.CHARGE_BLOCK : after(l_lowrateInterval-p_vPaceWidth,msec)
      VOOR.PACE.CHARGE_BLOCK -> VOOR.PACE.DISCHARGE_CHARGE : after(p_vPaceWidth,msec)
      VOOR.PACE.INIT_LRL -> VOOR.PACE.DISCHARGE_CHARGE
      (default) -> VOOR.PACE.INIT_LRL
    state SETTER [parallel]
      settings: executionOrder=2
      note: the status of the
          | setpoint is reevaluated
          | every 100 msec
      note: if the lowrateInterval is much lower than the setpoint,
          | it is incremented in INC_INT
      state INC_INT
        entry:
        l_lowrateInterval=l_lowrateInterval+10;
      state CHECK_SET
      state STAY
      note: if the lowrateInterval is negligibly close to the
          | setpoint, nothing is changed
      state DEC_INT
        entry:
        l_lowrateInterval=l_lowrateInterval-10;
      note: if the lowrateInterval is much higher than the setpoint,
          | it is decremented in DEC_INT
      (default) -> VOOR.SETTER.CHECK_SET
      VOOR.SETTER.INC_INT -> VOOR.SETTER.CHECK_SET : after(100,msec)
      (junction 457) -> VOOR.SETTER.INC_INT [order 2] : [l_setpoint-10>l_lowrateInterval]
      VOOR.SETTER.CHECK_SET -> (junction 457) [order 1] : [l_setpoint+10>=l_lowrateInterval]
      (junction 457) -> VOOR.SETTER.STAY [order 1] : [l_setpoint-10<=l_lowrateInterval]
      VOOR.SETTER.DEC_INT -> VOOR.SETTER.CHECK_SET : after(100,msec)
      VOOR.SETTER.STAY -> VOOR.SETTER.CHECK_SET : after(100,msec)
      VOOR.SETTER.CHECK_SET -> VOOR.SETTER.DEC_INT [order 2] : [l_setpoint+10<l_lowrateInterval]
    state TIMER [parallel]
      settings: executionOrder=4
      note: value of l_status (the number of recent acceleration spikes) is checked every 3 seconds,
          | and a setpoint is assigned accordingly
      note: the priority of the state transition arrows ensures that only one setpoint is used.
      state PICK_ACTIVITY
      state REST
        entry:
        l_setpoint=1000;
      state SPRINT
        entry:
        l_setpoint=330;
      state F_JOG
        entry:
        l_setpoint=425;
      state F_WALK
        entry:
        l_setpoint=600;
      state RESET_TIME
        entry:
        l_status=0;
      state RUN
        entry:
        l_setpoint=375;
      state S_JOG
        entry:
        l_setpoint=500;
      state S_WALK
        entry:
        l_setpoint=750;
      note: resets l_status
          | for each loop
      state END_TIME
      VOOR.TIMER.RESET_TIME -> VOOR.TIMER.PICK_ACTIVITY : after(3000,msec)
      VOOR.TIMER.PICK_ACTIVITY -> VOOR.TIMER.SPRINT [order 1] : [l_status>=7]
      VOOR.TIMER.PICK_ACTIVITY -> VOOR.TIMER.RUN [order 2] : [l_status>=6]
      VOOR.TIMER.PICK_ACTIVITY -> VOOR.TIMER.F_JOG [order 3] : [l_status>=5]
      VOOR.TIMER.PICK_ACTIVITY -> VOOR.TIMER.S_JOG [order 4] : [l_status>=4]
      VOOR.TIMER.PICK_ACTIVITY -> VOOR.TIMER.F_WALK [order 5] : [l_status>=3]
      VOOR.TIMER.PICK_ACTIVITY -> VOOR.TIMER.S_WALK [order 6] : [l_status>=2]
      VOOR.TIMER.PICK_ACTIVITY -> VOOR.TIMER.REST [order 7] : [l_status<2]
      (default) -> VOOR.TIMER.RESET_TIME
      VOOR.TIMER.REST -> VOOR.TIMER.END_TIME
      VOOR.TIMER.SPRINT -> VOOR.TIMER.END_TIME
      VOOR.TIMER.F_JOG -> VOOR.TIMER.END_TIME
      VOOR.TIMER.F_WALK -> VOOR.TIMER.END_TIME
      VOOR.TIMER.END_TIME -> VOOR.TIMER.RESET_TIME
      VOOR.TIMER.RUN -> VOOR.TIMER.END_TIME
      VOOR.TIMER.S_JOG -> VOOR.TIMER.END_TIME
      VOOR.TIMER.S_WALK -> VOOR.TIMER.END_TIME
    state COUNTER [parallel]
      settings: executionOrder=3
      note: increments l_status if acceleration passes a threshold
      state BLANK
      state ADD_COUNT
        entry:
        l_status=l_status+1;
      note: delay represents the maximum expected
          | width of the acceleration spike
          | (prevents multiple increments for 1 spike)
      (default) -> VOOR.COUNTER.BLANK
      VOOR.COUNTER.BLANK -> VOOR.COUNTER.ADD_COUNT : [r_accel>=2]
      VOOR.COUNTER.ADD_COUNT -> VOOR.COUNTER.BLANK : after(200,msec)
  state AOOR
    state PACE [parallel]
      settings: executionOrder=1
      state DISCHARGE_CHARGE
        entry:
        PACING_REF_PWM=p_aPaceAmp;
        PACE_CHARGE_CTRL=true;
        ATR_PACE_CTRL=false;
        ATR_GND_CTRL=true;
        PACE_GND_CTRL=true;
        GREEN_LED = false;
        RED_LED = false;
      state CHARGE_BLOCK
        entry:
        PACE_CHARGE_CTRL=false;
        ATR_PACE_CTRL=true;
        ATR_GND_CTRL=false;
        GREEN_LED = true;
      state INIT_LRL
        entry:
        l_lowrateInterval=p_lowrateInterval;
        l_setpoint = l_lowrateInterval;
      AOOR.PACE.DISCHARGE_CHARGE -> AOOR.PACE.CHARGE_BLOCK : after(l_lowrateInterval-p_aPaceWidth,msec)
      AOOR.PACE.CHARGE_BLOCK -> AOOR.PACE.DISCHARGE_CHARGE : after(p_aPaceWidth,msec)
      AOOR.PACE.INIT_LRL -> AOOR.PACE.DISCHARGE_CHARGE
      (default) -> AOOR.PACE.INIT_LRL
    state SETTER [parallel]
      settings: executionOrder=2
      state INC_INT
        entry:
        l_lowrateInterval=l_lowrateInterval+10;
      state CHECK_SET
      state STAY
      state DEC_INT
        entry:
        l_lowrateInterval=l_lowrateInterval-10;
      (default) -> AOOR.SETTER.CHECK_SET
      AOOR.SETTER.INC_INT -> AOOR.SETTER.CHECK_SET : after(100,msec)
      (junction 594) -> AOOR.SETTER.INC_INT [order 2] : [l_setpoint-10>l_lowrateInterval]
      AOOR.SETTER.CHECK_SET -> (junction 594) [order 1] : [l_setpoint+10>=l_lowrateInterval]
      (junction 594) -> AOOR.SETTER.STAY [order 1] : [l_setpoint-10<=l_lowrateInterval]
      AOOR.SETTER.DEC_INT -> AOOR.SETTER.CHECK_SET : after(100,msec)
      AOOR.SETTER.STAY -> AOOR.SETTER.CHECK_SET : after(100,msec)
      AOOR.SETTER.CHECK_SET -> AOOR.SETTER.DEC_INT [order 2] : [l_setpoint+10<l_lowrateInterval]
    state TIMER [parallel]
      settings: executionOrder=4
      state PICK_ACTIVITY
      state REST
        entry:
        l_setpoint=1000;
      state SPRINT
        entry:
        l_setpoint=330;
      state F_JOG
        entry:
        l_setpoint=425;
      state F_WALK
        entry:
        l_setpoint=600;
      state RESET_TIME
        entry:
        l_status=0;
      state RUN
        entry:
        l_setpoint=375;
      state S_JOG
        entry:
        l_setpoint=500;
      state S_WALK
        entry:
        l_setpoint=750;
      state END_TIME
      AOOR.TIMER.RESET_TIME -> AOOR.TIMER.PICK_ACTIVITY : after(3000,msec)
      AOOR.TIMER.PICK_ACTIVITY -> AOOR.TIMER.SPRINT [order 1] : [l_status>=7]
      AOOR.TIMER.PICK_ACTIVITY -> AOOR.TIMER.RUN [order 2] : [l_status>=6]
      AOOR.TIMER.PICK_ACTIVITY -> AOOR.TIMER.F_JOG [order 3] : [l_status>=5]
      AOOR.TIMER.PICK_ACTIVITY -> AOOR.TIMER.S_JOG [order 4] : [l_status>=4]
      AOOR.TIMER.PICK_ACTIVITY -> AOOR.TIMER.F_WALK [order 5] : [l_status>=3]
      AOOR.TIMER.PICK_ACTIVITY -> AOOR.TIMER.S_WALK [order 6] : [l_status>=2]
      AOOR.TIMER.PICK_ACTIVITY -> AOOR.TIMER.REST [order 7] : [l_status<2]
      (default) -> AOOR.TIMER.RESET_TIME
      AOOR.TIMER.REST -> AOOR.TIMER.END_TIME
      AOOR.TIMER.SPRINT -> AOOR.TIMER.END_TIME
      AOOR.TIMER.F_JOG -> AOOR.TIMER.END_TIME
      AOOR.TIMER.F_WALK -> AOOR.TIMER.END_TIME
      AOOR.TIMER.END_TIME -> AOOR.TIMER.RESET_TIME
      AOOR.TIMER.RUN -> AOOR.TIMER.END_TIME
      AOOR.TIMER.S_JOG -> AOOR.TIMER.END_TIME
      AOOR.TIMER.S_WALK -> AOOR.TIMER.END_TIME
    state COUNTER [parallel]
      settings: executionOrder=3
      state BLANK
      state ADD_COUNT
        entry:
        l_status=l_status+1;
      (default) -> AOOR.COUNTER.BLANK
      AOOR.COUNTER.BLANK -> AOOR.COUNTER.ADD_COUNT : [r_accel>=2]
      AOOR.COUNTER.ADD_COUNT -> AOOR.COUNTER.BLANK : after(200,msec)
    note: identical to VOOR (left) except atrial variables are used instead
  (default) -> CHOOSE_MODE
  CHOOSE_MODE -> VOO [order 5] : [p_mode==5]
  VOO -> CHOOSE_MODE : [p_mode~=5]
  CHOOSE_MODE -> VVIR [order 1] : [p_mode==14]
  CHOOSE_MODE -> AOO [order 4] : [p_mode==3]
  VVIR -> CHOOSE_MODE : [p_mode~=14]
  AOO -> CHOOSE_MODE : [p_mode~=3]
  VVI -> CHOOSE_MODE : [p_mode~=6]
  CHOOSE_MODE -> VVI [order 6] : [p_mode==6]
  CHOOSE_MODE -> AAIR [order 2] : [p_mode==12]
  AAIR -> CHOOSE_MODE : [p_mode~=12]
  AAI -> CHOOSE_MODE : [p_mode~=4]
  CHOOSE_MODE -> AAI [order 3] : [p_mode==4]
  CHOOSE_MODE -> AOOR [order 8] : [p_mode ==11]
  VOOR -> CHOOSE_MODE : [p_mode~=13]
  AOOR -> CHOOSE_MODE : [p_mode~=11]
  CHOOSE_MODE -> VOOR [order 7] : [p_mode==13]
  data: p_vPaceWidth input uint16; l_status local uint16; l_lowrateInterval local uint16; p_aPaceWidth input uint16; p_VRP input uint16; p_ARP input uint16; p_lowrateInterval input uint16; p_vPaceAmp input double; p_aPaceAmp input double; p_mode input uint8; r_accel input double; PACE_CHARGE_CTRL output boolean; VENT_CMP_REF_PWM output double; PACING_REF_PWM output double; ATR_CMP_REF_PWM output double; ATR_PACE_CTRL output boolean; VENT_PACE_CTRL output boolean; PACE_GND_CTRL output boolean; ATR_GND_CTRL output boolean; VENT_GND_CTRL output boolean; FRONTEND_CTRL output boolean; l_setpoint local uint16; GREEN_LED output boolean; RED_LED output boolean; BLUE_LED output boolean; spontPace input boolean; VENT_CMP_DETECT input boolean; ATR_CMP_DETECT input boolean; l_paced local boolean; l_sense local boolean
